simulink library "Damper_Control_None"  (R2023b)
settings: Solver=VariableStepAuto  StartTime=0.0  StopTime=10.0  RelTol=1e-3
libraries: Vehicle_Outputs x1
Description:
  | Copyright 2026 The MathWorks, Inc.
settings Model: Creator=smiller  LastModifiedBy=smiller
settings OptimizationCC: ReuseModelBlockBuffer=off
settings ModelReferenceCC: EnableRefExpFcnMdlSchedulingChecks=on

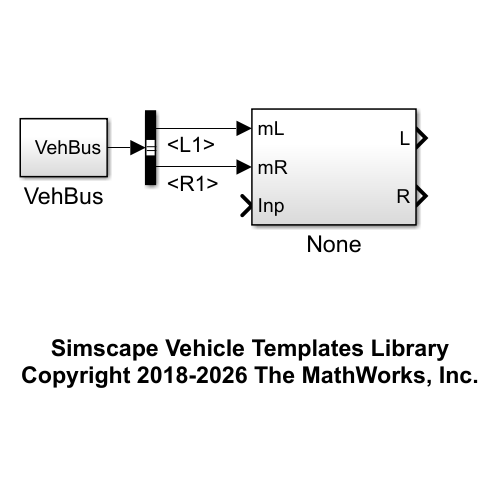
[thumbnail: Simulink's stored preview of the top-level diagram]
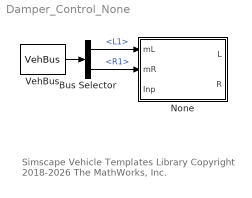
== system Damper_Control_None ==
  note: Simscape Vehicle Templates Library
      | Copyright 2018-2026 The MathWorks, Inc.
  Bus Selector : BusSelector  OutputSignals=Chassis.Damper.L1,Chassis.Damper.R1
  None : Subsystem  VariantControl=Choice
  VehBus : Vehicle_Outputs/VehBus  SystemSampleTime=-1  VariantActivationTime=update diagram  AllowFlexibleInterface=on  Latency=0  AutoFrameSizeCalculation=off
  wires:
  VehBus/1 -> Bus Selector/1
  Bus Selector/1 -> None/1(mL)  "<L1>"
  Bus Selector/2 -> None/2(mR)  "<R1>"

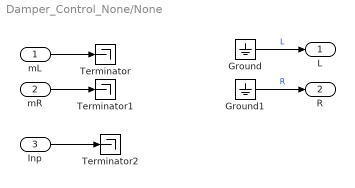
== system Damper_Control_None/None ==
  mL : Inport
  mR : Inport  Port=2
  Inp : Inport  Port=3
  Ground : Ground
  Ground1 : Ground
  Terminator : Terminator
  Terminator1 : Terminator
  Terminator2 : Terminator
  L : Outport  VectorParamsAs1DForOutWhenUnconnected=off
  R : Outport  Port=2  VectorParamsAs1DForOutWhenUnconnected=off
  wires:
  Ground/1 -> L/1  "L"
  Ground1/1 -> R/1  "R"
  mL/1 -> Terminator/1
  mR/1 -> Terminator1/1
  Inp/1 -> Terminator2/1
